simulink model "cps_slider_processor_v2"  (R2012b)
settings: Solver=FixedStepDiscrete  StartTime=0.0  StopTime=8.5  RelTol=20e-5
model workspace (MAT data in the model file):
  ini_block_hpos = -0.4
  ini_block_vpos = 0.11
  ini_nozzle_vpos = 0.3
undefined symbols (not defined in the file or in its folder): f
libraries: simulink x3
settings Model: Creator=pmosterm  LastModifiedBy=pmosterm
settings SolverCC: ZcThreshold=2e-5  MaxConsecutiveZCs=20  EnableConcurrentExecution=on  ConcurrentTasks=on  ZeroCrossAlgorithm=Adaptive  SolverResetMethod=Robust
settings DataIOCC: SignalLoggingSaveFormat=ModelDataLogs
settings OptimizationCC: InlineParams=on
settings DebuggingCC: AlgebraicLoopMsg=error  UnderspecifiedInitializationDetection=Simplified  FcnCallInpInsideContextMsg=EnableAllAsWarning  ModelReferenceExtraNoncontSigs=warning
settings ModelReferenceCC: ModelReferenceNumInstancesAllowed=Single
settings GRTTargetCC: CombineOutputUpdateFcns=off  GRTInterface=on
settings ConfigurationSet: Description=SimMechanics 2G

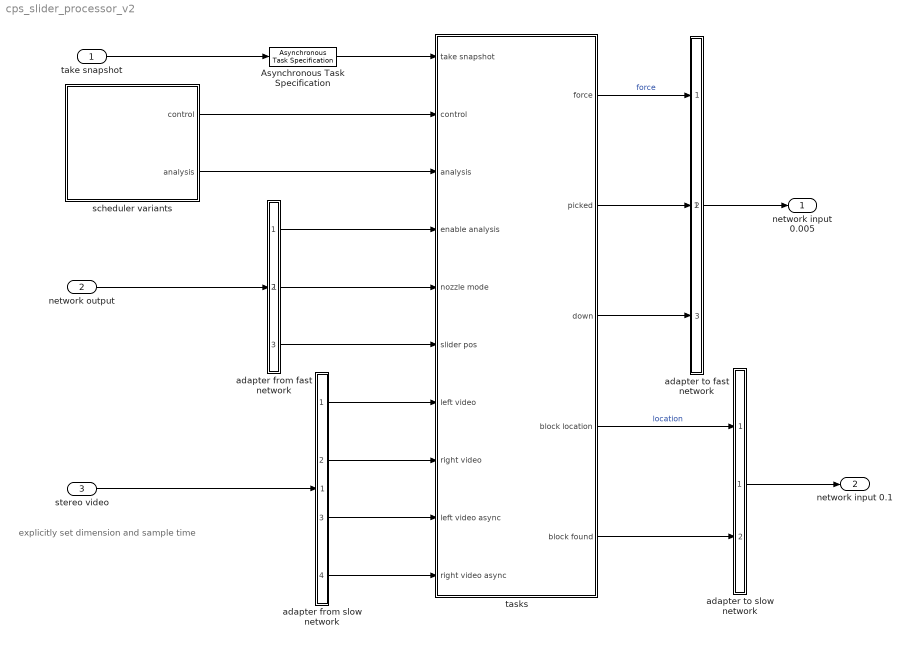
== system cps_slider_processor_v2 ==
  note: explicitly set dimension
      | and sample time
  take snapshot : Inport  OutputFunctionCall=on
  network output : Inport  Port=2  OutDataTypeStr=Bus: slBusSliderControlOps
  stereo video : Inport  Port=3  PortDimensions=[400 240 6]  SampleTime=0.1
  Asynchronous Task Specification : AsynchronousTaskSpecification  TaskPriority=5
  adapter from fast network : Subsystem
      mask Display: color('black');
  adapter from slow network : Subsystem
      mask Display: color('black');
  adapter to fast network : Subsystem
      mask Display: color('black');
  adapter to slow network : Subsystem
      mask Display: color('black');
  scheduler variants : Subsystem  Variant=on  OverrideUsingVariant=singlerate
  tasks : Subsystem
  network input 0.005 : Outport  OutDataTypeStr=Bus: slBusNozzleControl  BusOutputAsStruct=on
  network input 0.1 : Outport  Port=2  OutDataTypeStr=Bus: slBusStereoOps  BusOutputAsStruct=on
  wires:
  take snapshot/1 -> Asynchronous Task Specification/1
  Asynchronous Task Specification/1 -> tasks/1(take snapshot)
  scheduler variants/2(analysis) -> tasks/3(analysis)
  scheduler variants/1(control) -> tasks/2(control)
  tasks/1(force) -> adapter to fast network/1(force)  "force"
  tasks/2(picked) -> adapter to fast network/2(picked)
  tasks/3(down) -> adapter to fast network/3(down)
  adapter to fast network/1(nozzle control) -> network input 0.005/1
  tasks/4(block location) -> adapter to slow network/1(location)  "location"
  tasks/5(block found) -> adapter to slow network/2(found)
  adapter to slow network/1(stereopsis operations) -> network input 0.1/1
  network output/1 -> adapter from fast network/1(slider control operations)
  adapter from fast network/1(stereo analysis enabled) -> tasks/4(enable analysis)
  adapter from fast network/2(nozzle mode) -> tasks/5(nozzle mode)
  adapter from fast network/3(slider position) -> tasks/6(slider pos)
  stereo video/1 -> adapter from slow network/1(stereo video stream)
  adapter from slow network/1(left video stream) -> tasks/7(left video)
  adapter from slow network/2(right video stream) -> tasks/8(right video)
  adapter from slow network/3(left video stream async) -> tasks/9(left video async)
  adapter from slow network/4(right video stream async) -> tasks/10(right video async)

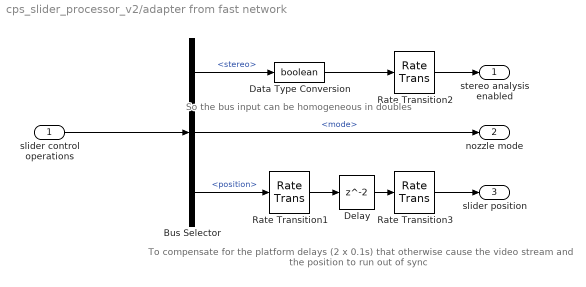
== system cps_slider_processor_v2/adapter from fast network ==
  note: So the bus input can be
      | homogeneous in doubles
  note: To compensate for the platform delays (2 x 0.1s)
      | that otherwise cause the video stream and the
      | position to run out of sync
  slider control operations : Inport
  Bus Selector : BusSelector  OutputSignals=stereo,mode,position
  Data Type Conversion : DataTypeConversion  OutDataTypeStr=boolean
  Delay : Delay  SampleTime=0.1
  Rate Transition1 : RateTransition  Deterministic=off
  Rate Transition2 : RateTransition  Deterministic=off
  Rate Transition3 : RateTransition  Deterministic=off
  stereo analysis enabled : Outport
  nozzle mode : Outport  Port=2
  slider position : Outport  Port=3
  wires:
  Bus Selector/1 -> Data Type Conversion/1  "<stereo>"
  Data Type Conversion/1 -> Rate Transition2/1
  Bus Selector/3 -> Rate Transition1/1  "<position>"
  Bus Selector/2 -> nozzle mode/1  "<mode>"
  Rate Transition2/1 -> stereo analysis enabled/1
  Rate Transition3/1 -> slider position/1
  slider control operations/1 -> Bus Selector/1
  Delay/1 -> Rate Transition3/1
  Rate Transition1/1 -> Delay/1

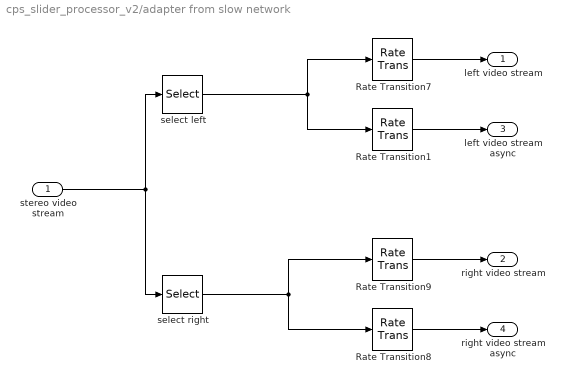
== system cps_slider_processor_v2/adapter from slow network ==
  stereo video stream : Inport
  Rate Transition{1,7..9} (4 alike) : RateTransition  Deterministic=off
  select left : Selector  NumberOfDimensions=3  InputPortWidth=3  IndexOptions=Select all,Select all,Index vector (dialog)  Indices=[1:400],1,1:3  OutputSizes=1,1,1
  select right : Selector  NumberOfDimensions=3  InputPortWidth=3  IndexOptions=Select all,Select all,Index vector (dialog)  Indices=[1:400],1,4:6  OutputSizes=1,1,1
  left video stream : Outport
  right video stream : Outport  Port=2
  left video stream async : Outport  Port=3
  right video stream async : Outport  Port=4
  wires:
  stereo video stream/1 -> select left/1, select right/1
  select right/1 -> Rate Transition9/1, Rate Transition8/1
  select left/1 -> Rate Transition1/1, Rate Transition7/1
  Rate Transition9/1 -> right video stream/1
  Rate Transition7/1 -> left video stream/1
  Rate Transition8/1 -> right video stream async/1
  Rate Transition1/1 -> left video stream async/1

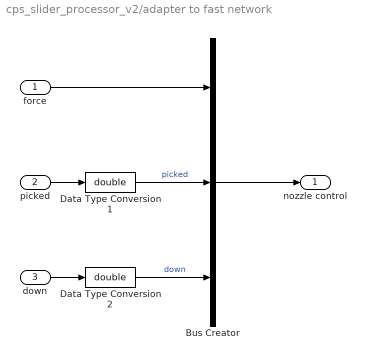
== system cps_slider_processor_v2/adapter to fast network ==
  force : Inport
  picked : Inport  Port=2
  down : Inport  Port=3
  Bus Creator : BusCreator  Inputs=3
  Data Type Conversion1 : DataTypeConversion  OutDataTypeStr=double
  Data Type Conversion2 : DataTypeConversion  OutDataTypeStr=double
  nozzle control : Outport
  wires:
  force/1 -> Bus Creator/1
  Data Type Conversion2/1 -> Bus Creator/3  "down"
  Bus Creator/1 -> nozzle control/1
  picked/1 -> Data Type Conversion1/1
  down/1 -> Data Type Conversion2/1
  Data Type Conversion1/1 -> Bus Creator/2  "picked"

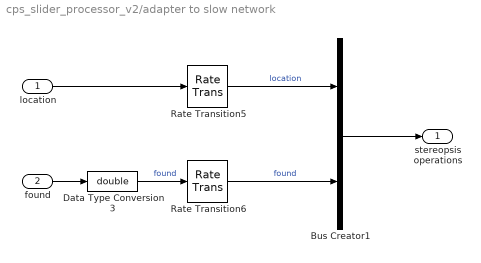
== system cps_slider_processor_v2/adapter to slow network ==
  location : Inport
  found : Inport  Port=2
  Bus Creator1 : BusCreator  Inputs='location','found'  OutDataTypeStr=Bus: slBusStereoOps
  Data Type Conversion3 : DataTypeConversion  OutDataTypeStr=double
  Rate Transition5 : RateTransition  Deterministic=off  OutPortSampleTime=0.1
  Rate Transition6 : RateTransition  Deterministic=off  OutPortSampleTime=0.1
  stereopsis operations : Outport
  wires:
  Bus Creator1/1 -> stereopsis operations/1
  location/1 -> Rate Transition5/1
  Rate Transition5/1 -> Bus Creator1/1  "location"
  Rate Transition6/1 -> Bus Creator1/2  "found"
  found/1 -> Data Type Conversion3/1
  Data Type Conversion3/1 -> Rate Transition6/1  "found"

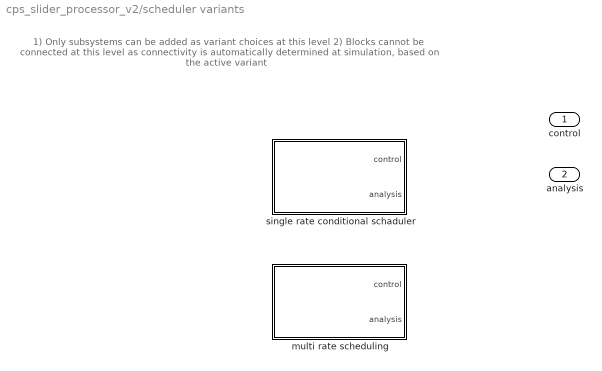
== system cps_slider_processor_v2/scheduler variants ==
  note: 1) Only subsystems can be added as variant choices at this level
      | 2) Blocks cannot be connected at this level as connectivity is
      | automatically determined at simulation, based on the active variant
  multi rate scheduling : Subsystem  VariantObject=multirate
  single rate conditional schaduler : Subsystem  VariantObject=singlerate
  control : Outport
  analysis : Outport  Port=2

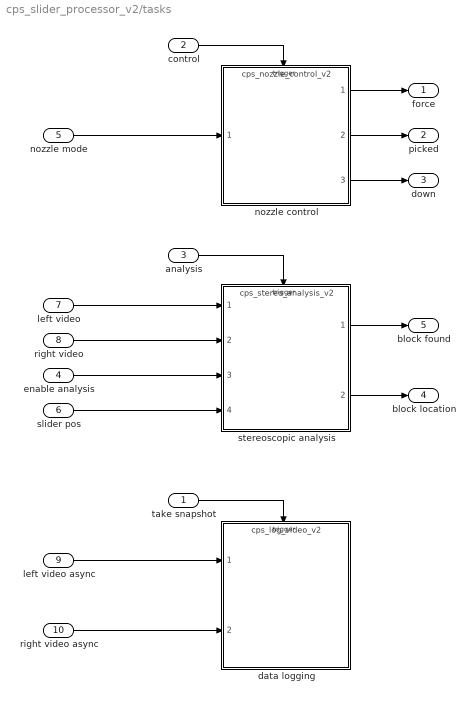
== system cps_slider_processor_v2/tasks ==
  take snapshot : Inport  OutputFunctionCall=on
  control : Inport  Port=2
  analysis : Inport  Port=3
  enable analysis : Inport  Port=4
  nozzle mode : Inport  Port=5
  slider pos : Inport  Port=6
  left video : Inport  Port=7
  right video : Inport  Port=8
  left video async : Inport  Port=9
  right video async : Inport  Port=10
  data logging : ModelReference  RequirementInfo={} %GIDa_3b488b36_65e4_448c_9ba9_b184886c03df  ModelNameDialog=cps_log_video_v2  SimulationMode=Normal  ModelReferenceVersion=1.564  CopyOfModelName=cps_log_video_v2  DefaultDataLogging=on  TriggerPortName=function  TriggerPortTriggerType=function-call  TriggerPortStatesWhenEnabling=held
  nozzle control : ModelReference  RequirementInfo={} %GIDa_87509e0b_fc0d_4efa_8955_ff7852c43de9  ModelNameDialog=cps_nozzle_control_v2  SimulationMode=Normal  ModelReferenceVersion=1.159  CopyOfModelName=cps_nozzle_control_v2  DefaultDataLogging=on  TriggerPortName=f()  TriggerPortTriggerType=function-call  TriggerPortStatesWhenEnabling=held
  stereoscopic analysis : ModelReference  ModelNameDialog=cps_stereo_analysis_v2  SimulationMode=Normal  Variant=on  ModelReferenceVersion=1.204  CopyOfModelName=cps_stereo_analysis_v2  DefaultDataLogging=on  TriggerPortName=f()  TriggerPortTriggerType=function-call  TriggerPortStatesWhenEnabling=held
      settings: AttributesFormatString=%<ActiveVariant>
  force : Outport
  picked : Outport  Port=2
  down : Outport  Port=3
  block location : Outport  Port=4
  block found : Outport  Port=5
  wires:
  nozzle mode/1 -> nozzle control/1
  nozzle control/1 -> force/1
  nozzle control/2 -> picked/1
  nozzle control/3 -> down/1
  right video/1 -> stereoscopic analysis/2
  left video/1 -> stereoscopic analysis/1
  stereoscopic analysis/2 -> block location/1
  stereoscopic analysis/1 -> block found/1
  take snapshot/1 -> data logging/Trigger
  enable analysis/1 -> stereoscopic analysis/3
  control/1 -> nozzle control/Trigger
  analysis/1 -> stereoscopic analysis/Trigger
  left video async/1 -> data logging/1
  right video async/1 -> data logging/2
  slider pos/1 -> stereoscopic analysis/4

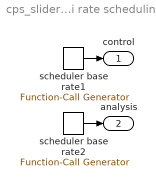
== system cps_slider_processor_v2/scheduler variants/multi rate scheduling ==
  scheduler base rate1 : simulink/Ports & Subsystems/Function-Call Generator  sample_time=0.005  numberOfIterations=1
  scheduler base rate2 : simulink/Ports & Subsystems/Function-Call Generator  sample_time=0.1  numberOfIterations=1
  control : Outport
  analysis : Outport  Port=2
  wires:
  scheduler base rate1/1 -> control/1
  scheduler base rate2/1 -> analysis/1

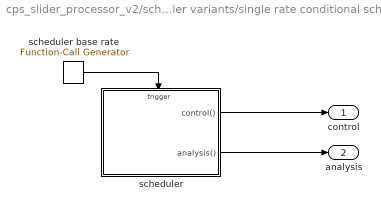
== system cps_slider_processor_v2/scheduler variants/single rate conditional schaduler ==
  scheduler : Stateflow chart  TreatAsAtomicUnit=on
  scheduler base rate : simulink/Ports & Subsystems/Function-Call Generator  sample_time=0.005  numberOfIterations=1
  control : Outport
  analysis : Outport  Port=2
  wires:
  scheduler base rate/1 -> scheduler/Trigger
  scheduler/1(control()) -> control/1
  scheduler/2(analysis()) -> analysis/1

== stateflow chart cps_slider_processor_v2/scheduler variants/single rate conditional schaduler/scheduler ==
  state scheduler
    state OneTick [parallel]
      on every(1,tick):
      control;
      settings: executionOrder=2
    state TenTick [parallel]
      on every(20,tick):
      control; analysis;
      settings: executionOrder=1
  (default) -> scheduler : /control; analysis;
  events: control output FUNCTION_CALL_EVENT; analysis output FUNCTION_CALL_EVENT; tick input FUNCTION_CALL_EVENT
